simulink model "OAC_LA_Ass1_Task2_simu"  (R2018a)
settings: Solver=VariableStepAuto  StartTime=0.0  StopTime=10.0  MaxStep=10e-3  RelTol=1e-3
values from neighbouring files (symbols this model uses):
  g = 9.81    [OAC_LA_Ass1.m]    (also in OAC_LA_Ass1_Task1.m; OAC_LA_Ass1_Task2.m)
  l = l_L1    [OAC_LA_Ass1.m]    (also in OAC_LA_Ass1_Task1.m = g/phat; OAC_LA_Ass1_Task2.m = 0.3; Task1_Funcs.m = g/phat)
  opt_params = params_Linfty    [OAC_LA_Ass1_Task2.m]
  x0 = [0; 0; 0; 0]    [OAC_LA_Ass1.m]    (also in OAC_LA_Ass1_Task2.m = [x_W(1); phi(1); v_W(1); omega(1)])
settings Model: Creator=miko2  LastModifiedBy=miko2

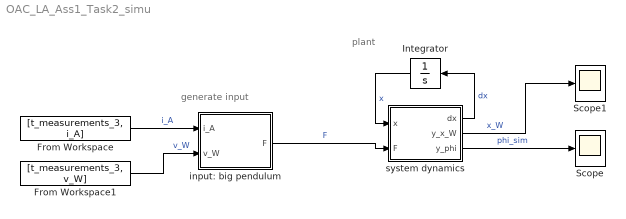
== system OAC_LA_Ass1_Task2_simu ==
  note: generate input
  note: plant
  From Workspace : FromWorkspace  VariableName=[t_measurements_3, i_A]  SampleTime=0
  From Workspace1 : FromWorkspace  VariableName=[t_measurements_3, v_W]  SampleTime=0
  Integrator : Integrator  InitialCondition=x0
  Scope : Scope
  Scope1 : Scope
  input: big pendulum : MATLAB Function  TreatAsAtomicUnit=on
  system dynamics : MATLAB Function  TreatAsAtomicUnit=on
  wires:
  system dynamics/3(y_phi) -> Scope/1  "phi_sim"
  Integrator/1 -> system dynamics/1(x)  "x"
  input: big pendulum/1(F) -> system dynamics/2(F)  "F"
  From Workspace/1 -> input: big pendulum/1(i_A)  "i_A"
  From Workspace1/1 -> input: big pendulum/2(v_W)  "v_W"
  system dynamics/1(dx) -> Integrator/1  "dx"
  system dynamics/2(y_x_W) -> Scope1/1  "x_W"

== matlab function OAC_LA_Ass1_Task2_simu/input: big pendulum ==
  data: i_A input; v_W input; F output; opt_params parameter
function F = fcn(i_A, v_W, opt_params)
    
    V = opt_params(3);
    k1 = opt_params(4);

    F = V*i_A - k1*v_W;

end

== matlab function OAC_LA_Ass1_Task2_simu/system dynamics ==
  data: dx output; x input; y_x_W output; F input; y_phi output; opt_params parameter; l parameter; g parameter
function [dx, y_x_W, y_phi] = fcn(x,F,opt_params,l,g)

    ms = opt_params(1);
    mw = opt_params(2);
    
    x_W = x(1);
    phi = x(2);
    v_W = x(3);
    omega = x(4);

    dx_W = v_W;
    dphi = omega;
    dv_W = 1/( mw + ms*(1-(cos(phi))^2) ) * ( F + ms*l*omega^2*sin(phi) ...
        - ms*g*sin(phi)*cos(phi) );
    domega = 1/( l * ( 1 - ms/(mw+ms)*(cos(phi))^2 ) ) * ( g*sin(phi) - ...
        cos(phi)/(ms+mw)*F - ms/(mw+ms)*l*omega^2*sin(phi)*cos(phi) );
    
    dx = [dx_W; dphi; dv_W; domega]; 
          
    y_x_W = x_W;
    y_phi = phi;

end
